simulink model "TiltCopter_TOSTO_v2"  (R2015a)
settings: Solver=ode45  StartTime=0.0  StopTime=10  RelTol=1e-3
values from neighbouring files (symbols this model uses):
  Fx = 0    [Main_tiltCopter_TOSTO.m]    (also in Main_tiltCopter_TOSTO_v2.m)
  Fy = 0    [Main_tiltCopter_TOSTO.m]    (also in Main_tiltCopter_TOSTO_v2.m = 0.2)
  U = [-1; 0; 0; 0]    [Main_tiltCopter_TOSTO.m]    (also in Main_tiltCopter_TOSTO_v2.m = [-1; 0; 0;0])
undefined symbols (not defined in the file or in its folder): b, B0, B1, B2, B3, degtorad, dLMN, g, I_Pi, In, InInv, KaD, KaI, KaN, KaP, Kba, Kbp, Kbq, Kbr, Kdp, Kdq, Kdr, Kip, Kiq, Kir, KPD, KPI, KPP, Kpp, Kpq, Kpr, Kq, KRD, KRI, KRP, Kt, m, m_servo, Mb, MbInv, N, omega_hover, pitchMax, q_servo, rollMax, satp, satq, satr, ServoMotor_Gain, tau, x1, yawRateMax
libraries: aerolibutil x10, simulink x6
(part 2 of 2)

== system TiltCopter_TOSTO_v2/TiltCopter/Actuators/External Momentum_1/Thrust computation ==
  omega_i : Inport
  Constant : Constant  Value=-Kt
  Constant1 : Constant  Value=0
  Constant2 : Constant  Value=0
  Mux : Mux  Inputs=3
  Product : Product
  Product1 : Product
  Vector_Thrust_i : Outport
  wires:
  Constant2/1 -> Mux/2
  omega_i/1 -> Product/2, Product/1
  Product/1 -> Product1/1
  Constant1/1 -> Mux/1
  Mux/1 -> Vector_Thrust_i/1
  Product1/1 -> Mux/3
  Constant/1 -> Product1/2

== system TiltCopter_TOSTO_v2/TiltCopter/Actuators/External Momentum_2/Thrust computation ==
  omega_i : Inport
  Constant : Constant  Value=-Kt
  Constant1 : Constant  Value=0
  Constant2 : Constant  Value=0
  Mux : Mux  Inputs=3
  Product : Product
  Product1 : Product
  Vector_Thrust_i : Outport
  wires:
  Constant2/1 -> Mux/2
  omega_i/1 -> Product/2, Product/1
  Product/1 -> Product1/1
  Constant1/1 -> Mux/1
  Mux/1 -> Vector_Thrust_i/1
  Product1/1 -> Mux/3
  Constant/1 -> Product1/2

== system TiltCopter_TOSTO_v2/TiltCopter/Actuators/External Momentum_3/Thrust computation ==
  omega_i : Inport
  Constant : Constant  Value=-Kt
  Constant1 : Constant  Value=0
  Constant2 : Constant  Value=0
  Mux : Mux  Inputs=3
  Product : Product
  Product1 : Product
  Vector_Thrust_i : Outport
  wires:
  Constant2/1 -> Mux/2
  omega_i/1 -> Product/2, Product/1
  Product/1 -> Product1/1
  Constant1/1 -> Mux/1
  Mux/1 -> Vector_Thrust_i/1
  Product1/1 -> Mux/3
  Constant/1 -> Product1/2

== system TiltCopter_TOSTO_v2/TiltCopter/Actuators/External Momentum_4/Thrust computation ==
  omega_i : Inport
  Constant : Constant  Value=-Kt
  Constant1 : Constant  Value=0
  Constant2 : Constant  Value=0
  Mux : Mux  Inputs=3
  Product : Product
  Product1 : Product
  Vector_Thrust_i : Outport
  wires:
  Constant2/1 -> Mux/2
  omega_i/1 -> Product/2, Product/1
  Product/1 -> Product1/1
  Constant1/1 -> Mux/1
  Mux/1 -> Vector_Thrust_i/1
  Product1/1 -> Mux/3
  Constant/1 -> Product1/2

== system TiltCopter_TOSTO_v2/TiltCopter/Actuators/Servo_Motor 1/Angle [rad] -> Pulse [ms] ==
  Pulse [ms] : Inport
  Add : Sum  Inputs=+-
  Constant : Constant  Value=q_servo
  Linear fitting gain : Gain  Gain=1/m_servo
  Angle [rad] : Outport
  wires:
  Constant/1 -> Add/2
  Add/1 -> Linear fitting gain/1
  Pulse [ms]/1 -> Add/1
  Linear fitting gain/1 -> Angle [rad]/1

== system TiltCopter_TOSTO_v2/TiltCopter/Actuators/Servo_Motor 2/Angle [rad] -> Pulse [ms] ==
  Pulse [ms] : Inport
  Add : Sum  Inputs=+-
  Constant : Constant  Value=q_servo
  Linear fitting gain : Gain  Gain=1/m_servo
  Angle [rad] : Outport
  wires:
  Constant/1 -> Add/2
  Add/1 -> Linear fitting gain/1
  Pulse [ms]/1 -> Add/1
  Linear fitting gain/1 -> Angle [rad]/1

== system TiltCopter_TOSTO_v2/TiltCopter/Actuators/Servo_Motor 3/Angle [rad] -> Pulse [ms] ==
  Pulse [ms] : Inport
  Add : Sum  Inputs=+-
  Constant : Constant  Value=q_servo
  Linear fitting gain : Gain  Gain=1/m_servo
  Angle [rad] : Outport
  wires:
  Constant/1 -> Add/2
  Add/1 -> Linear fitting gain/1
  Pulse [ms]/1 -> Add/1
  Linear fitting gain/1 -> Angle [rad]/1

== system TiltCopter_TOSTO_v2/TiltCopter/Actuators/Servo_Motor 4/Angle [rad] -> Pulse [ms] ==
  Pulse [ms] : Inport
  Add : Sum  Inputs=+-
  Constant : Constant  Value=q_servo
  Linear fitting gain : Gain  Gain=1/m_servo
  Angle [rad] : Outport
  wires:
  Constant/1 -> Add/2
  Add/1 -> Linear fitting gain/1
  Pulse [ms]/1 -> Add/1
  Linear fitting gain/1 -> Angle [rad]/1

== system TiltCopter_TOSTO_v2/TiltCopter/Actuators/Traslational Force_1/Thrust computation ==
  omega_i : Inport
  Constant : Constant  Value=-Kt
  Constant1 : Constant  Value=0
  Constant2 : Constant  Value=0
  Mux : Mux  Inputs=3
  Product : Product
  Product1 : Product
  Vector_Thrust_i : Outport
  wires:
  Constant2/1 -> Mux/2
  omega_i/1 -> Product/2, Product/1
  Product/1 -> Product1/1
  Constant1/1 -> Mux/1
  Mux/1 -> Vector_Thrust_i/1
  Product1/1 -> Mux/3
  Constant/1 -> Product1/2

== system TiltCopter_TOSTO_v2/TiltCopter/Actuators/Traslational Force_2/Thrust computation ==
  omega_i : Inport
  Constant : Constant  Value=-Kt
  Constant1 : Constant  Value=0
  Constant2 : Constant  Value=0
  Mux : Mux  Inputs=3
  Product : Product
  Product1 : Product
  Vector_Thrust_i : Outport
  wires:
  Constant2/1 -> Mux/2
  omega_i/1 -> Product/2, Product/1
  Product/1 -> Product1/1
  Constant1/1 -> Mux/1
  Mux/1 -> Vector_Thrust_i/1
  Product1/1 -> Mux/3
  Constant/1 -> Product1/2

== system TiltCopter_TOSTO_v2/TiltCopter/Actuators/Traslational Force_3/Thrust computation ==
  omega_i : Inport
  Constant : Constant  Value=-Kt
  Constant1 : Constant  Value=0
  Constant2 : Constant  Value=0
  Mux : Mux  Inputs=3
  Product : Product
  Product1 : Product
  Vector_Thrust_i : Outport
  wires:
  Constant2/1 -> Mux/2
  omega_i/1 -> Product/2, Product/1
  Product/1 -> Product1/1
  Constant1/1 -> Mux/1
  Mux/1 -> Vector_Thrust_i/1
  Product1/1 -> Mux/3
  Constant/1 -> Product1/2

== system TiltCopter_TOSTO_v2/TiltCopter/Actuators/Traslational Force_4/Thrust computation ==
  omega_i : Inport
  Constant : Constant  Value=-Kt
  Constant1 : Constant  Value=0
  Constant2 : Constant  Value=0
  Mux : Mux  Inputs=3
  Product : Product
  Product1 : Product
  Vector_Thrust_i : Outport
  wires:
  Constant2/1 -> Mux/2
  omega_i/1 -> Product/2, Product/1
  Product/1 -> Product1/1
  Constant1/1 -> Mux/1
  Mux/1 -> Vector_Thrust_i/1
  Product1/1 -> Mux/3
  Constant/1 -> Product1/2

== system TiltCopter_TOSTO_v2/TiltCopter/Actuators/tau_p1 computation/Drag torque computation ==
  omega_P1_z : Inport
  Constant : Constant  Value=-Kq
  Constant1 : Constant  Value=0
  Constant2 : Constant  Value=0
  Demux : Demux  Outputs=3
  Mux : Mux  Inputs=3
  Product : Product
  Product1 : Product
  Terminator : Terminator
  Terminator1 : Terminator
  Vector_DragTorque_i : Outport
  wires:
  Constant2/1 -> Mux/2
  Product/1 -> Product1/1
  Constant1/1 -> Mux/1
  Mux/1 -> Vector_DragTorque_i/1
  Product1/1 -> Mux/3
  Constant/1 -> Product1/2
  Demux/1 -> Terminator/1
  Demux/2 -> Terminator1/1
  omega_P1_z/1 -> Product/2, Product/1

== system TiltCopter_TOSTO_v2/TiltCopter/Actuators/tau_p2 computation/Drag torque computation ==
  omega_P2 : Inport
  Constant : Constant  Value=Kq
  Constant1 : Constant  Value=0
  Constant2 : Constant  Value=0
  Mux : Mux  Inputs=3
  Product : Product
  Product1 : Product
  Vector_DragTorque_i : Outport
  wires:
  Constant2/1 -> Mux/2
  Product/1 -> Product1/1
  Constant1/1 -> Mux/1
  Mux/1 -> Vector_DragTorque_i/1
  Product1/1 -> Mux/3
  Constant/1 -> Product1/2
  omega_P2/1 -> Product/2, Product/1

== system TiltCopter_TOSTO_v2/TiltCopter/Actuators/tau_p3 computation1/Drag torque computation ==
  omega_P3 : Inport
  Constant : Constant  Value=-Kq
  Constant1 : Constant  Value=0
  Constant2 : Constant  Value=0
  Demux : Demux  Outputs=3
  Mux : Mux  Inputs=3
  Product : Product
  Product1 : Product
  Terminator : Terminator
  Terminator1 : Terminator
  Vector_DragTorque_i : Outport
  wires:
  Constant2/1 -> Mux/2
  Product/1 -> Product1/1
  Constant1/1 -> Mux/1
  Mux/1 -> Vector_DragTorque_i/1
  Product1/1 -> Mux/3
  Constant/1 -> Product1/2
  Demux/1 -> Terminator/1
  Demux/2 -> Terminator1/1
  omega_P3/1 -> Product/2, Product/1

== system TiltCopter_TOSTO_v2/TiltCopter/Actuators/tau_p4 computation2/Drag torque computation ==
  omega_P4 : Inport
  Constant : Constant  Value=Kq
  Constant1 : Constant  Value=0
  Constant2 : Constant  Value=0
  Demux : Demux  Outputs=3
  Mux : Mux  Inputs=3
  Product : Product
  Product1 : Product
  Terminator : Terminator
  Terminator1 : Terminator
  Vector_DragTorque_i : Outport
  wires:
  Constant2/1 -> Mux/2
  Product/1 -> Product1/1
  Constant1/1 -> Mux/1
  Mux/1 -> Vector_DragTorque_i/1
  Product1/1 -> Mux/3
  Constant/1 -> Product1/2
  Demux/1 -> Terminator/1
  Demux/2 -> Terminator1/1
  omega_P4/1 -> Product/2, Product/1

== matlab function TiltCopter_TOSTO_v2/TiltCopter/To body from Earth ==
  data: Alpha_e input; Earth input; body output
 function body = Tbe(Alpha_e, Earth)
%#codegen
phi = Alpha_e(1);
theta = Alpha_e(2);
psi = Alpha_e(3);

Sphi = sin(phi);
Cphi = cos(phi);
Stheta = sin(theta);
Ctheta = cos(theta);
Spsi = sin(psi);
Cpsi = cos(psi);

TBE = [        Ctheta*Cpsi               Ctheta*Spsi          -Stheta    ;
       Sphi*Stheta*Cpsi-Cphi*Spsi Sphi*Stheta*Spsi+Cphi*Cpsi Sphi*Ctheta ;
       Cphi*Stheta*Cpsi+Sphi*Spsi Cphi*Stheta*Spsi-Sphi*Cpsi Cphi*Ctheta];

body = TBE* Earth;

== matlab function TiltCopter_TOSTO_v2/TiltCopter/To Earth from body ==
  data: Alpha_e input; Earth output; body input
 function Earth = Tbet(Alpha_e, body)
%#codegen
phi = Alpha_e(1);
theta = Alpha_e(2);
psi = Alpha_e(3);

Sphi = sin(phi);
Cphi = cos(phi);
Stheta = sin(theta);
Ctheta = cos(theta);
Spsi = sin(psi);
Cpsi = cos(psi);

TBE = [        Ctheta*Cpsi               Ctheta*Spsi          -Stheta    ;
       Sphi*Stheta*Cpsi-Cphi*Spsi Sphi*Stheta*Spsi+Cphi*Cpsi Sphi*Ctheta ;
       Cphi*Stheta*Cpsi+Sphi*Spsi Cphi*Stheta*Spsi-Sphi*Cpsi Cphi*Ctheta];
TEB = TBE';

Earth = TEB* body;

== matlab function TiltCopter_TOSTO_v2/TiltCopter/To Earth from body_rates ==
  data: Alpha_e input; Rates_B input; Rates_E output
 function Rates_E = Einv(Alpha_e, Rates_B)
%#codegen
phi = Alpha_e(1);
theta = Alpha_e(2);

Sphi = sin(phi);
Cphi = cos(phi);
Ctheta = cos(theta);
Ttheta = tan(theta);

Einv = [1   Sphi*Ttheta    Cphi*Ttheta ;
        0       Cphi          -Sphi    ;
        0   Sphi/Ctheta    Cphi/Ctheta];

Rates_E = Einv* Rates_B;

== matlab function TiltCopter_TOSTO_v2/TiltCopter/Actuators/Traslational Force_1/R_BP1 ==
  data: Rotation_matrix output; alpha_1 input
function Rotation_matrix = fcn(alpha_1)
%#codegen

% Rotation matrix from group propeller 1 to body
R_BP1 = [ 1,0,0; 0, cos(alpha_1), -sin(alpha_1);0, sin(alpha_1),cos(alpha_1)];
      



Rotation_matrix = R_BP1;

== matlab function TiltCopter_TOSTO_v2/Mixer Function/NONLINEAR mixer/Inverted NONLINEAR mixer matrix ==
  data: Fx input; Fy input; T input; L input; M input; N input; y output; omega_hover parameter; Kt parameter; Kq parameter; b parameter
function y = fcn(Fx,Fy,T,L,M,N,omega_hover,Kt,Kq,b)
%#codegen

omega_1 = omega_hover;
omega_2 = omega_hover;
omega_3 = omega_hover;
omega_4 = omega_hover;

% Calcolo prima gli alpha per ottenere la Fx e Fy desiderata considerando
% una omega di hovering
alpha_2 = -asin(Fx/(Kt*(omega_2^2 + omega_4^2)));

alpha_1 = asin(Fy/(Kt*(omega_1^2 + omega_3^2)));
alpha_3 = -alpha_1;
alpha_4 = -alpha_2;

% A questo punto risolvo la matrice K_mix, considerando gli angoli noti e
% risolvo solo per omega_i
K_mix = [
    -Kt*cos(alpha_1),                      -Kt*cos(alpha_2),                    -Kt*cos(alpha_3),                    -Kt*cos(alpha_4);
                                   0, - Kq*sin(alpha_2) - Kt*b*cos(alpha_2),                                   0, Kq*sin(alpha_4) + Kt*b*cos(alpha_4);
 Kt*b*cos(alpha_1) - Kq*sin(alpha_1),                                     0, Kq*sin(alpha_3) - Kt*b*cos(alpha_3),                                   0;
 Kq*cos(alpha_1) + Kt*b*sin(alpha_1),   Kt*b*sin(alpha_2) - Kq*cos(alpha_2), Kq*cos(alpha_3) + Kt*b*sin(alpha_3), Kt*b*sin(alpha_4) - Kq*cos(alpha_4)];

Omega_result = inv(K_mix)*[T;L;M;N];
y = [Omega_result;alpha_1;alpha_2;alpha_3;alpha_4];

== matlab function TiltCopter_TOSTO_v2/Controllers/Attitude Controller/To body from Earth_rates ==
  data: Alpha_e input; Rates_B output; Rates_E input
 function Rates_B = E(Alpha_e, Rates_E)
%#codegen
phi = Alpha_e(1);       % Roll
theta = Alpha_e(2);     % Pitch
psi = Alpha_e(3);       % Yaw

E = [cos(psi)*cos(theta),cos(theta)*sin(psi),-sin(theta);
 cos(psi)*sin(phi)*sin(theta) - cos(phi)*sin(psi), cos(phi)*cos(psi) + sin(phi)*sin(psi)*sin(theta), cos(theta)*sin(phi);
 sin(phi)*sin(psi) + cos(phi)*cos(psi)*sin(theta), cos(phi)*sin(psi)*sin(theta) - cos(psi)*sin(phi), cos(phi)*cos(theta)];

Rates_B = E* Rates_E;

== matlab function TiltCopter_TOSTO_v2/Mixer Function/NONLINEAR mixer/round1 ==
  data: u input; y output
function y = fcn(u)
%#codegen
 risultato = round(u*100)/100;
y = risultato;

== matlab function TiltCopter_TOSTO_v2/Mixer Function/NONLINEAR mixer/round2 ==
  data: u input; y output
function y = fcn(u)
%#codegen
 risultato = round(u*100)/100;
y = risultato;

== matlab function TiltCopter_TOSTO_v2/Mixer Function/NONLINEAR mixer/round3 ==
  data: u input; y output
function y = fcn(u)
%#codegen
 risultato = round(u*100)/100;
y = risultato;

== matlab function TiltCopter_TOSTO_v2/Mixer Function/NONLINEAR mixer/round4 ==
  data: u input; y output
function y = fcn(u)
%#codegen
 risultato = round(u*100)/100;
y = risultato;

== matlab function TiltCopter_TOSTO_v2/TiltCopter/Actuators/dOmega_Pi and Omega_Pi computation 1/Time Derivative R_P1B ==
  data: alpha_1 input; dalpha_1 input; Rotation_matrix output
function Rotation_matrix = fcn(alpha_1,dalpha_1)
%#codegen
dR_P1B = [ 0 0 0 ; 
          0 -sin(alpha_1) cos(alpha_1);
          0 -cos(alpha_1) -sin(alpha_1)];
      
Rotation_matrix = dR_P1B*dalpha_1;

== matlab function TiltCopter_TOSTO_v2/TiltCopter/Actuators/dOmega_Pi and Omega_Pi computation2/Time Derivative R_P2B ==
  data: alpha_2 input; dalpha_2 input; Rotation_matrix output
function Rotation_matrix = fcn(alpha_2,dalpha_2)
%#codegen
% omega_x = -dalpha_i;
% omega_y = 0;
% omega_z = 0;
% Define the skew simmetric matrix
% S = [0 -omega_z omega_y;omega_z 0 -omega_x; -omega_y omega_x 0];


%Time derivative of Rotation matrix from Body to propeller group 1
% This rotation matrix is obtained with the Skew symmetric matrix
% In fact R_dot = S(alpha) * R_BPi

dR_P2B = [ 0 0 0 ; sin(alpha_2) 0 cos(alpha_2);...
           cos(alpha_2) 0 -sin(alpha_2)];
      
Rotation_matrix = dR_P2B*dalpha_2;

== matlab function TiltCopter_TOSTO_v2/TiltCopter/Actuators/dOmega_Pi and Omega_Pi computation3/Time Derivative R_P3B ==
  data: alpha_3 input; dalpha_3 input; Rotation_matrix output
function Rotation_matrix = fcn(alpha_3,dalpha_3)
%#codegen
dR_P3B =[ 0 0 0 ; 0 sin(alpha_3) cos(alpha_3); 0 cos(alpha_3) -sin(alpha_3)]; 
      
Rotation_matrix = dR_P3B*dalpha_3;

== matlab function TiltCopter_TOSTO_v2/TiltCopter/Actuators/Traslational Force_2/R_BP2 ==
  data: Rotation_matrix output; alpha_2 input
function Rotation_matrix = fcn(alpha_2)
%#codegen

% Rotation matrix from Propeller group 2 to body
R_BP2 =[ 0, -cos(alpha_2), sin(alpha_2); 1,0,0; 0,sin(alpha_2),cos(alpha_2)];

Rotation_matrix =R_BP2;

== matlab function TiltCopter_TOSTO_v2/TiltCopter/Actuators/Traslational Force_3/R_BP3 ==
  data: Rotation_matrix output; alpha_3 input
function Rotation_matrix = fcn(alpha_3)
%#codegen

R_BP3 = [ -1, 0, 0;0, -cos(alpha_3), sin(alpha_3);0,  sin(alpha_3), cos(alpha_3)];

Rotation_matrix = R_BP3;

== matlab function TiltCopter_TOSTO_v2/TiltCopter/Actuators/Traslational Force_4/R_BP4 ==
  data: Rotation_matrix output; alpha_4 input
function Rotation_matrix = fcn(alpha_4)
%#codegen

R_BP4 = [0, cos(alpha_4), -sin(alpha_4); -1, 0, 0; 0, sin(alpha_4), cos(alpha_4)];

Rotation_matrix = R_BP4;

== matlab function TiltCopter_TOSTO_v2/TiltCopter/Actuators/dOmega_Pi and Omega_Pi computation4/Time Derivative R_P4B ==
  data: alpha_4 input; dalpha_4 input; Rotation_matrix output
function Rotation_matrix = fcn(alpha_4,dalpha_4)
%#codegen
dR_P4B = [ 0 0 0 ; -sin(alpha_4) 0 cos(alpha_4); -cos(alpha_4) 0 -sin(alpha_4)];
Rotation_matrix = dR_P4B*dalpha_4;

== matlab function TiltCopter_TOSTO_v2/TiltCopter/Actuators/External Momentum_1/O_BPi ==
  data: Origin_Rotation output; motor_number input; b parameter
function Origin_Rotation = fcn(motor_number,b)
%#codegen

% Rotation matrix from Body to propeller group
psi = (motor_number-1)*pi/2;


R_z = [cos(psi), -sin(psi), 0;
      sin(psi),  cos(psi), 0;
      0,         0, 1];
      



Origin_Rotation = R_z*[b;0;0];

== matlab function TiltCopter_TOSTO_v2/TiltCopter/Actuators/External Momentum_1/R_BP1 ==
  data: Rotation_matrix output; alpha_1 input
function Rotation_matrix = fcn(alpha_1)
%#codegen

% Rotation matrix from group propeller 1 to body
R_BP1 = [ 1,0,0; 0, cos(alpha_1), -sin(alpha_1);0, sin(alpha_1),cos(alpha_1)];
      



Rotation_matrix = R_BP1;

== matlab function TiltCopter_TOSTO_v2/TiltCopter/Actuators/External Momentum_2/O_BPi ==
  data: Origin_Rotation output; motor_number input; b parameter
function Origin_Rotation = fcn(motor_number,b)
%#codegen

% Rotation matrix from Body to propeller group
psi = (motor_number-1)*pi/2;


R_z =[ cos(psi), -sin(psi), 0;
      sin(psi),  cos(psi), 0;
      0,         0, 1];
      



Origin_Rotation = R_z*[b;0;0];

== matlab function TiltCopter_TOSTO_v2/TiltCopter/Actuators/External Momentum_2/R_BP2 ==
  data: Rotation_matrix output; alpha_2 input
function Rotation_matrix = fcn(alpha_2)
%#codegen

% Rotation matrix from Propeller group 2 to body
R_BP2 =[ 0, -cos(alpha_2), sin(alpha_2); 1,0,0; 0,sin(alpha_2),cos(alpha_2)];

Rotation_matrix =R_BP2;

== matlab function TiltCopter_TOSTO_v2/TiltCopter/Actuators/External Momentum_3/O_BPi ==
  data: Origin_Rotation output; motor_number input; b parameter
function Origin_Rotation = fcn(motor_number,b)
%#codegen

% Rotation matrix from Body to propeller group
psi = (motor_number-1)*pi/2;


R_z = [cos(psi), -sin(psi), 0;
      sin(psi),  cos(psi), 0;
      0,         0, 1];
      



Origin_Rotation = R_z*[b;0;0];

== matlab function TiltCopter_TOSTO_v2/TiltCopter/Actuators/External Momentum_3/R_BP3 ==
  data: Rotation_matrix output; alpha_3 input
function Rotation_matrix = fcn(alpha_3)
%#codegen

R_BP3 = [ -1, 0, 0;0, -cos(alpha_3), sin(alpha_3);0,  sin(alpha_3), cos(alpha_3)];

Rotation_matrix = R_BP3;

== matlab function TiltCopter_TOSTO_v2/TiltCopter/Actuators/External Momentum_4/O_BPi ==
  data: Origin_Rotation output; motor_number input; b parameter
function Origin_Rotation = fcn(motor_number,b)
%#codegen

% Rotation matrix from Body to propeller group
psi = (motor_number-1)*pi/2;


R_z = [cos(psi), -sin(psi), 0;
      sin(psi),  cos(psi), 0;
      0,         0, 1];
      



Origin_Rotation = R_z*[b;0;0];

== matlab function TiltCopter_TOSTO_v2/TiltCopter/Actuators/External Momentum_4/R_BP4 ==
  data: Rotation_matrix output; alpha_4 input
function Rotation_matrix = fcn(alpha_4)
%#codegen

R_BP4 = [0, cos(alpha_4), -sin(alpha_4); -1, 0, 0; 0, sin(alpha_4), cos(alpha_4)];

Rotation_matrix = R_BP4;

== matlab function TiltCopter_TOSTO_v2/TiltCopter/Actuators/dOmega_Pi and Omega_Pi computation2/R_P2B ==
  data: alpha_2 input; Rotation_matrix output
function Rotation_matrix = fcn(alpha_2)
%#codegen
R_P2B = [0 1 0; -cos(alpha_2) 0 sin(alpha_2);sin(alpha_2) 0 cos(alpha_2)];
      
Rotation_matrix = R_P2B;

== matlab function TiltCopter_TOSTO_v2/TiltCopter/Actuators/dOmega_Pi and Omega_Pi computation3/R_P3B ==
  data: alpha_3 input; Rotation_matrix output
function Rotation_matrix = fcn(alpha_3)
%#codegen
R_P3B = [ -1 0 0 ; 0 -cos(alpha_3) sin(alpha_3); 0 sin(alpha_3) cos(alpha_3)];
      
Rotation_matrix = R_P3B;

== matlab function TiltCopter_TOSTO_v2/TiltCopter/Actuators/dOmega_Pi and Omega_Pi computation 1/R_P1B ==
  data: alpha_1 input; Rotation_matrix output
function Rotation_matrix = fcn(alpha_1)
%#codegen
R_P1B = [ 1 0 0 ; 0 cos(alpha_1) sin(alpha_1); 0 -sin(alpha_1) cos(alpha_1)];
      
Rotation_matrix = R_P1B;

== matlab function TiltCopter_TOSTO_v2/TiltCopter/Actuators/dOmega_Pi and Omega_Pi computation4/R_P4B ==
  data: alpha_4 input; Rotation_matrix output
function Rotation_matrix = fcn(alpha_4)
%#codegen
R_P4B = [0 -1 0; cos(alpha_4) 0 sin(alpha_4); -sin(alpha_4) 0 cos(alpha_4)];
      
Rotation_matrix = R_P4B;

== matlab function TiltCopter_TOSTO_v2/TiltCopter/Actuators/dOmega_Pi and Omega_Pi computation2/R_P2B1 ==
  data: alpha_2 input; Rotation_matrix output
function Rotation_matrix = fcn(alpha_2)
%#codegen
R_P2B = [0 1 0; -cos(alpha_2) 0 sin(alpha_2);sin(alpha_2) 0 cos(alpha_2)];
      
Rotation_matrix = R_P2B;

== matlab function TiltCopter_TOSTO_v2/TiltCopter/Actuators/dOmega_Pi and Omega_Pi computation3/R_P3B1 ==
  data: alpha_3 input; Rotation_matrix output
function Rotation_matrix = fcn(alpha_3)
%#codegen
R_P3B = [ -1 0 0 ; 0 -cos(alpha_3) sin(alpha_3); 0 sin(alpha_3) cos(alpha_3)];
      
Rotation_matrix = R_P3B;

== matlab function TiltCopter_TOSTO_v2/TiltCopter/Actuators/dOmega_Pi and Omega_Pi computation4/R_P4B1 ==
  data: alpha_4 input; Rotation_matrix output
function Rotation_matrix = fcn(alpha_4)
%#codegen
R_P4B = [0 -1 0; cos(alpha_4) 0 sin(alpha_4); -sin(alpha_4) 0 cos(alpha_4)];
      
Rotation_matrix = R_P4B;
